simulink model "VVI_STATE"  (R2020a)
settings: Solver=FixedStepAuto  StartTime=0.0  StopTime=10.0  FixedStep=1e-3  RelTol=1e-3  EnableMultiTasking=on
undefined symbols (not defined in the file): D1, D10, D12, D13, D2, D3, D5, D7, D9, PTA1, PTA2, PTB9, PTC17, PTC3, PTC4, PTD0, PTD1, PTD3
libraries: frdmk64flib x11
settings Model: ExtModeTrigDuration=5  Creator=ishap  LastModifiedBy=ishap
settings OptimizationCC: EnhancedBackFolding=on  PassReuseOutputArgsAs=Individual arguments  ZeroExternalMemoryAtStartup=off  ZeroInternalMemoryAtStartup=off  MaxStackSize=64  OptimizeBlockOrder=speed  DifferentSizesBufferReuse=on  OptimizationCustomize=off  EfficientTunableParamExpr=on
settings DebuggingCC: ParameterTunabilityLossMsg=error
settings HardwareCC: ProdBitPerPointer=32  ProdBitPerSizeT=32  ProdBitPerPtrDiffT=32  ProdLargestAtomicInteger=Long  ProdLargestAtomicFloat=Double  ProdWordSize=32  ProdHWDeviceType=ARM Compatible->ARM Cortex
settings SFSimCC: MATLABDynamicMemAlloc=off
settings RTWCC: SystemTargetFile=ert.tlc  HardwareBoard=NXP FRDM-K64F  TemplateMakefile=ert_default_tmf  Toolchain=GNU Tools for ARM Embedded Processors
settings CodeAppCC: ForceParamTrailComments=on  IgnoreCustomStorageClasses=off  OperatorAnnotations=on  SimulinkDataObjDesc=on  SFDataObjDesc=on  InsertBlockDesc=on

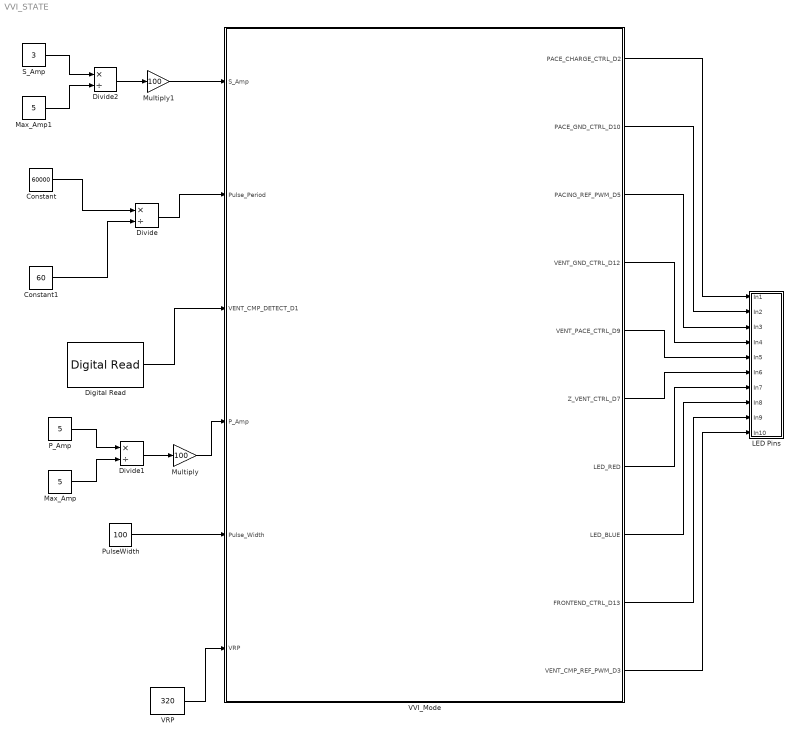
== system VVI_STATE ==
  Constant : Constant  Value=60000
  Constant1 : Constant  Value=60
  Digital Read : frdmk64flib/Digital Read  Whichpin=PTC17 (D1)  SampleTime=-1
  Divide : Product  Inputs=*/
  Divide1 : Product  Inputs=*/
  Divide2 : Product  Inputs=*/
  LED Pins : Subsystem
  Max_Amp : Constant  Value=5
  Max_Amp1 : Constant  Value=5
  Multiply : Gain  Gain=100
  Multiply1 : Gain  Gain=100
  P_Amp : Constant  Value=5
  PulseWidth : Constant  Value=100
  S_Amp : Constant  Value=3
  VRP : Constant  Value=320
  VVI_Mode : Stateflow chart  TreatAsAtomicUnit=on
      settings: PortSchema="{\"entries\":[{\"content\":{\"sides\":[{\"content\":{\"connectorIds\":[\"In1\",\"In2\",\"In3\",\"In5\",\"In4\",\"In6\"]},\"type\":\"ConnectorPlacement.EquallySpacedRectSide\",\"uuid\":\"7f50778c-a42a-4ed4-9c61-e38bb863925f\"},{\"content\":{\"connectorIds\":[\"Out1\",\"Out2\",\"Out3\",\"Out4\",\"Out5\",\"Out6\",\"Out7\",\"Out8\",\"Out9\",\"Out10\"],\"side\":\"RIGHT\"},\"type\":\"ConnectorPlacement.EquallySpacedRectSide\",\"uuid\":\"dafd7489-8283-4586-bb80-e827392d4a6f\"},{\"content\":{\"connectorIds\":[],\"side\":\"TOP\"},\"type\":\"ConnectorPlacement.EquallySpacedRectSide\",\"uuid\":\"186793bc-f9e1-404e-b87c-fd8bda3ef417\"}]},\"type\":\"ConnectorPlacement.EquallySpacedConnector\",\"uuid\":\"380b3cf5-cd26-4912-a10d-15eb89f6f210\"}],\"packageUris\":[\"http://schema.mathworks.com/mf0/Connector/19700101\"],\"version\":\"1.0\"}"
  wires:
  VRP/1 -> VVI_Mode/6(VRP)
  Constant/1 -> Divide/1
  Constant1/1 -> Divide/2
  Divide/1 -> VVI_Mode/2(Pulse_Period)
  VVI_Mode/1(PACE_CHARGE_CTRL_D2) -> LED Pins/1(In1)
  VVI_Mode/2(PACE_GND_CTRL_D10) -> LED Pins/2(In2)
  VVI_Mode/3(PACING_REF_PWM_D5) -> LED Pins/3(In3)
  VVI_Mode/4(VENT_GND_CTRL_D12) -> LED Pins/4(In4)
  VVI_Mode/5(VENT_PACE_CTRL_D9) -> LED Pins/5(In5)
  VVI_Mode/6(Z_VENT_CTRL_D7) -> LED Pins/6(In6)
  VVI_Mode/7(LED_RED) -> LED Pins/7(In7)
  VVI_Mode/8(LED_BLUE) -> LED Pins/8(In8)
  VVI_Mode/9(FRONTEND_CTRL_D13) -> LED Pins/9(In9)
  VVI_Mode/10(VENT_CMP_REF_PWM_D3) -> LED Pins/10(In10)
  Digital Read/1 -> VVI_Mode/3(VENT_CMP_DETECT_D1)
  PulseWidth/1 -> VVI_Mode/4(Pulse_Width)
  P_Amp/1 -> Divide1/1
  Max_Amp/1 -> Divide1/2
  Divide1/1 -> Multiply/1
  Multiply/1 -> VVI_Mode/5(P_Amp)
  Max_Amp1/1 -> Divide2/2
  Divide2/1 -> Multiply1/1
  S_Amp/1 -> Divide2/1
  Multiply1/1 -> VVI_Mode/1(S_Amp)

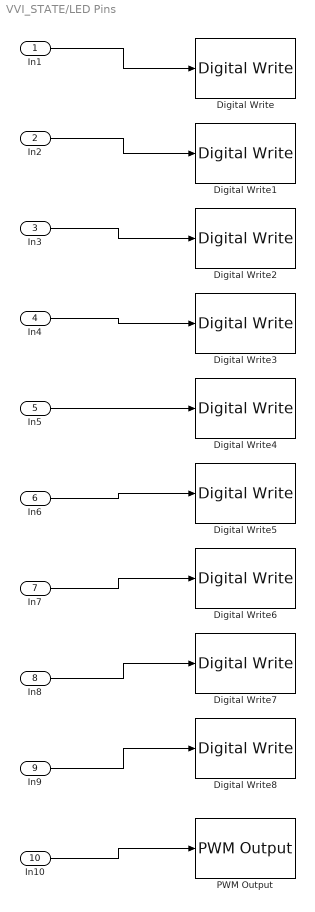
== system VVI_STATE/LED Pins ==
  In1 : Inport
  In2 : Inport  Port=2
  In3 : Inport  Port=3
  In4 : Inport  Port=4
  In5 : Inport  Port=5
  In6 : Inport  Port=6
  In7 : Inport  Port=7
  In8 : Inport  Port=8
  In9 : Inport  Port=9
  In10 : Inport  Port=10
  Digital Write : frdmk64flib/Digital Write  Whichpin=PTB9 (D2)
  Digital Write1 : frdmk64flib/Digital Write  Whichpin=PTD0 (D10)
  Digital Write2 : frdmk64flib/Digital Write  Whichpin=PTA2 (D5)
  Digital Write3 : frdmk64flib/Digital Write  Whichpin=PTD3 (D12)
  Digital Write4 : frdmk64flib/Digital Write  Whichpin=PTC4 (D9)
  Digital Write5 : frdmk64flib/Digital Write  Whichpin=PTC3 (D7)
  Digital Write6 : frdmk64flib/Digital Write  Whichpin=RED_LED
  Digital Write7 : frdmk64flib/Digital Write  Whichpin=BLUE_LED
  Digital Write8 : frdmk64flib/Digital Write  Whichpin=PTD1 (D13)
  PWM Output : frdmk64flib/PWM Output  Whichpin=PTA1 (D3)  InitialFrequency=2000  InitialDutyCycle=0
  wires:
  In4/1 -> Digital Write3/1
  In5/1 -> Digital Write4/1
  In6/1 -> Digital Write5/1
  In8/1 -> Digital Write7/1
  In1/1 -> Digital Write/1
  In7/1 -> Digital Write6/1
  In2/1 -> Digital Write1/1
  In10/1 -> PWM Output/1
  In9/1 -> Digital Write8/1
  In3/1 -> Digital Write2/1

== stateflow chart VVI_STATE/VVI_Mode ==
  state Pacing
    entry:
    PACING_REF_PWM_D5 = P_Amp;
    PACE_CHARGE_CTRL_D2 = 0;
    VENT_PACE_CTRL_D9 = 1;
    VENT_GND_CTRL_D12 = 0;
    PACE_GND_CTRL_D10 = 1;
    Z_VENT_CTRL_D7 = 0;
    LED_RED = 1;
    LED_BLUE = 0;
  state Charge_and_Sense
    entry:
    FRONTEND_CTRL_D13 = 1;
    PACING_REF_PWM_D5 = P_Amp;
    VENT_CMP_REF_PWM_D3 = S_Amp;
    PACE_CHARGE_CTRL_D2 = 1;
    VENT_PACE_CTRL_D9 = 0;
    VENT_GND_CTRL_D12 = 1;
    PACE_GND_CTRL_D10 = 0;
    Z_VENT_CTRL_D7 = 0;
    LED_RED = 0;
    LED_BLUE = 1;
  (default) -> Charge_and_Sense
  (junction 22) -> Charge_and_Sense [order 1] : [VENT_CMP_DETECT_D1 == 1]
  Charge_and_Sense -> (junction 22) : [after(VRP-Pulse_Width,msec)]
  (junction 22) -> Pacing [order 2] : after(Pulse_Period- VRP,msec)[VENT_CMP_DETECT_D1 == 0]
  Pacing -> Charge_and_Sense : [after(Pulse_Width,msec)]
  data: S_Amp input; Pulse_Period input; VENT_CMP_DETECT_D1 input; Pulse_Width input; P_Amp input; PACE_CHARGE_CTRL_D2 output; PACE_GND_CTRL_D10 output; PACING_REF_PWM_D5 output; VENT_GND_CTRL_D12 output; VENT_PACE_CTRL_D9 output; Z_VENT_CTRL_D7 output; LED_RED output; LED_BLUE output; FRONTEND_CTRL_D13 output; VENT_CMP_REF_PWM_D3 output; VRP input
